simulink model "leg"  (R2024a)
settings: Solver=ode15s  StartTime=0.0  StopTime=11  FixedStep=0.1  RelTol=1e-3
values from neighbouring files (symbols this model uses):
  m = RIGHT_LEG(joint_name).m    [test_dynamics.m]
  motion_time_constant = 1e-3    (= 0.001)    [Initialization.m]
undefined symbols (not defined in the file or in its folder): LEFT_LEG_FEEDBACK_GAIN, RIGHT_LEG_FEEDBACK_GAIN, X, Y, Z
libraries: sm_lib x104, nesl_utility x35, slpidlib x20
(part 1 of 5)
settings Model: Creator=daniel  LastModifiedBy=daniel

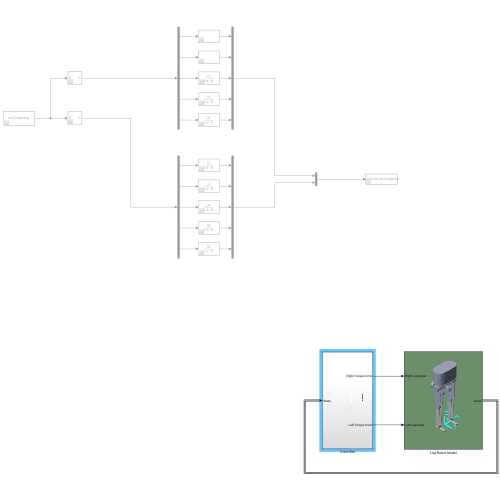
[thumbnail: Simulink's stored preview of the top-level diagram]
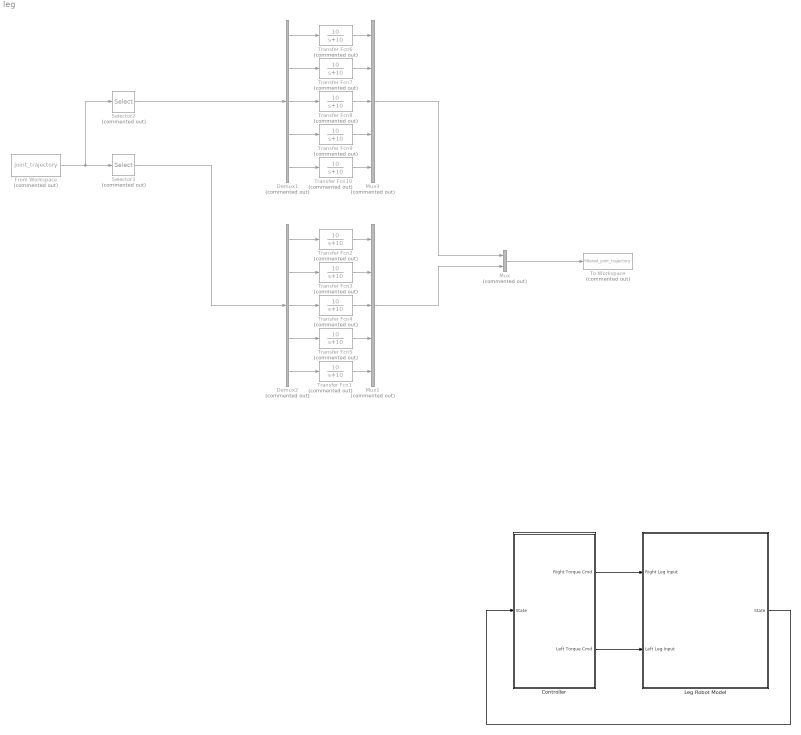
== system leg ==
  Controller : Subsystem
  Demux1 : Demux  Commented=on  Outputs=5
  Demux2 : Demux  Commented=on  Outputs=5
  From Workspace : FromWorkspace  Commented=on  VariableName=joint_trajectory
  Leg Robot Model : Subsystem
      mask Display: image('leg_robot.png');
  Mux : Mux  Commented=on  Inputs=2
  Mux1 : Mux  Commented=on  Inputs=5
  Mux3 : Mux  Commented=on  Inputs=5
  Selector2 : Selector  Commented=on  InputPortWidth=10  IndexOptions=Index vector (dialog)  Indices=[1:5]  OutputSizes=1
  Selector3 : Selector  Commented=on  InputPortWidth=10  IndexOptions=Index vector (dialog)  Indices=[6:10]  OutputSizes=1
  To Workspace : ToWorkspace  Commented=on  VariableName=filtered_joint_trajectory  SaveFormat=Structure With Time  SampleTime=-1
  Transfer Fcn{1..10} (10 alike) : TransferFcn  Commented=on  Numerator=[10]  Denominator=[1 10]
  wires:
  Controller/1(Right Torque Cmd) -> Leg Robot Model/1(Right Leg Input)
  Controller/2(Left Torque Cmd) -> Leg Robot Model/2(Left Leg Input)
  Leg Robot Model/1(State) -> Controller/1(State)
  Transfer Fcn10/1 -> Mux3/5
  Demux1/5 -> Transfer Fcn10/1
  Demux1/3 -> Transfer Fcn8/1
  Transfer Fcn6/1 -> Mux3/1
  Demux1/4 -> Transfer Fcn9/1
  Transfer Fcn8/1 -> Mux3/3
  Transfer Fcn7/1 -> Mux3/2
  Transfer Fcn9/1 -> Mux3/4
  Demux1/1 -> Transfer Fcn6/1
  Demux1/2 -> Transfer Fcn7/1
  From Workspace/1 -> Selector2/1, Selector3/1
  Selector2/1 -> Demux1/1
  Selector3/1 -> Demux2/1
  Transfer Fcn4/1 -> Mux1/3
  Transfer Fcn2/1 -> Mux1/1
  Demux2/5 -> Transfer Fcn1/1
  Transfer Fcn3/1 -> Mux1/2
  Demux2/2 -> Transfer Fcn3/1
  Mux1/1 -> Mux/2
  Demux2/4 -> Transfer Fcn5/1
  Transfer Fcn5/1 -> Mux1/4
  Demux2/1 -> Transfer Fcn2/1
  Demux2/3 -> Transfer Fcn4/1
  Transfer Fcn1/1 -> Mux1/5
  Mux/1 -> To Workspace/1
  Mux3/1 -> Mux/1

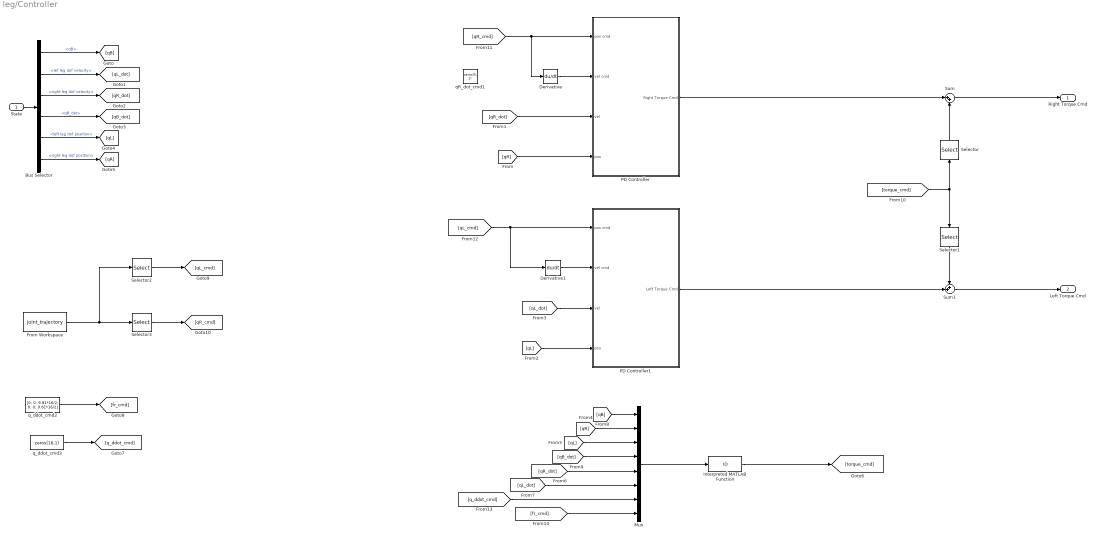
== system leg/Controller ==
  State : Inport
  Bus Selector : BusSelector  OutputSignals=qB,lef leg dof velocity,right leg dof velocity,qB_dot,left leg dof position,right leg dof position
  Derivative : Derivative  CoefficientInTFapproximation=0
  Derivative1 : Derivative  CoefficientInTFapproximation=0
  From Workspace : FromWorkspace  VariableName=joint_trajectory
  Interpreted MATLAB Function : MATLABFcn  MATLABFcn=ID
  Mux : Mux  Inputs=8
  PD Controller : Subsystem
  PD Controller1 : Subsystem
  Selector : Selector  InputPortWidth=10  IndexOptions=Index vector (dialog)  Indices=[1:5]  OutputSizes=1
  Selector1 : Selector  InputPortWidth=10  IndexOptions=Index vector (dialog)  Indices=[6:10]  OutputSizes=1
  Selector2 : Selector  InputPortWidth=10  IndexOptions=Index vector (dialog)  Indices=[1:5]  OutputSizes=1
  Selector3 : Selector  InputPortWidth=10  IndexOptions=Index vector (dialog)  Indices=[6:10]  OutputSizes=1
  Sum : Sum  Inputs=|++
  Sum1 : Sum  Inputs=++|
  qR_dot_cmd1 : Constant  Value=zeros(5, 1)
  q_ddot_cmd2 : Constant  Value=[0; 0; 9.81*16/2; 0; 0; 9.81*16/2]
  q_ddot_cmd3 : Constant  Value=zeros(16,1)
  Right Torque Cmd : Outport
  Left Torque Cmd : Outport  Port=2
  wires:
  State/1 -> Bus Selector/1
  Bus Selector/1 -> [qB]  "<qB>"
  Bus Selector/2 -> [qL_dot]  "<lef leg dof velocity>"
  Bus Selector/3 -> [qR_dot]  "<right leg dof velocity>"
  Bus Selector/4 -> [qB_dot]  "<qB_dot>"
  Bus Selector/5 -> [qL]  "<left leg dof position>"
  Bus Selector/6 -> [qR]  "<right leg dof position>"
  [qR] -> PD Controller/4(pos)
  [qR_dot] -> PD Controller/3("vel ")
  [qL] -> PD Controller1/4(pos)
  [qL_dot] -> PD Controller1/3("vel ")
  PD Controller/1(Right Torque Cmd) -> Sum/1
  Sum/1 -> Right Torque Cmd/1
  Sum1/1 -> Left Torque Cmd/1
  PD Controller1/1(Left Torque Cmd) -> Sum1/2
  Selector/1 -> Sum/2
  Selector1/1 -> Sum1/1
  [q_ddot_cmd] -> Mux/7
  [qL] -> Mux/3
  [qR] -> Mux/2
  [qL_dot] -> Mux/6
  [qR_dot] -> Mux/5
  [qB] -> Mux/1
  [qB_dot] -> Mux/4
  [fr_cmd] -> Mux/8
  [torque_cmd] -> Selector1/1, Selector/1
  Mux/1 -> Interpreted MATLAB Function/1
  From Workspace/1 -> Selector3/1, Selector2/1
  Selector2/1 -> [qL_cmd]
  Selector3/1 -> [qR_cmd]
  q_ddot_cmd2/1 -> [fr_cmd]
  q_ddot_cmd3/1 -> [q_ddot_cmd]
  Derivative/1 -> PD Controller/2(vel cmd)
  Derivative1/1 -> PD Controller1/2(vel cmd)
  Interpreted MATLAB Function/1 -> [torque_cmd]
  [qL_cmd] -> Derivative1/1, PD Controller1/1(pos cmd)
  [qR_cmd] -> Derivative/1, PD Controller/1(pos cmd)

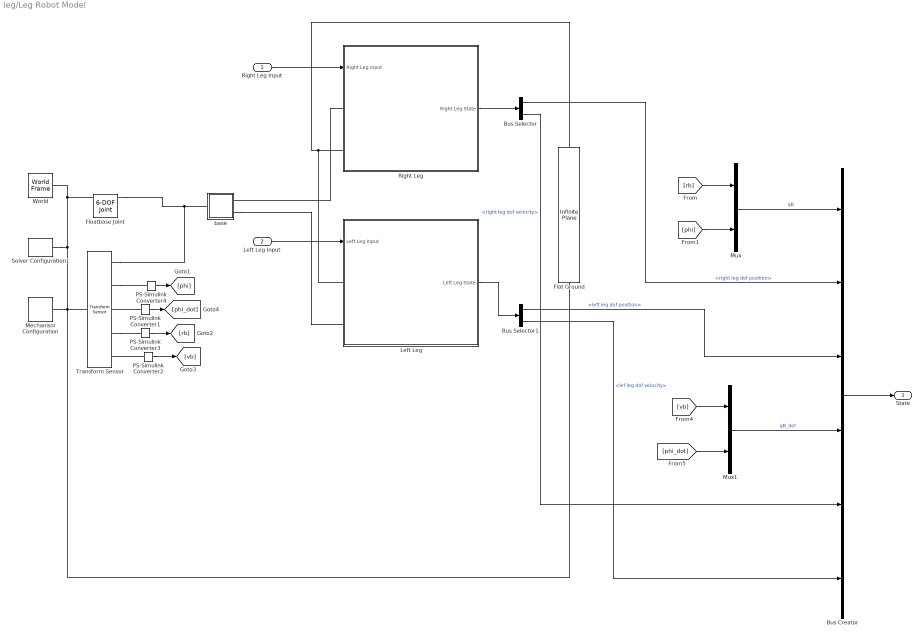
== system leg/Leg Robot Model ==
  Right Leg Input : Inport
  Left Leg Input : Inport  Port=2
  Bus Creator : BusCreator  Inputs=6
  Bus Selector : BusSelector  OutputSignals=right leg dof position,right leg dof velocity
  Bus Selector1 : BusSelector  OutputSignals=left leg dof position,lef leg dof velocity
  Flat Ground : sm_lib/Curves and Surfaces/Infinite Plane  GraphicType=Rectangle  GraphicPlaneWidth=5  GraphicPlaneWidthUnits=m  GraphicPlaneHeight=5  GraphicPlaneHeightUnits=m  GraphicVisPropType=SimpleVisualProperties  GraphicDiffuseColor=[0.07451 0.6235 1]  GraphicOpacity=0.75  GraphicSpecularColor=[0.5 0.5 0.5 1.0]  GraphicAmbientColor=[0.15 0.15 0.15 1.0]  GraphicEmissiveColor=[0.0 0.0 0.0 1.0]  GraphicShininess=75
  Floatbase Joint : sm_lib/Joints/6-DOF Joint  JointMode=Normal  CompositeWrenchDir=FollowerOnBase  CompositeWrenchFrame=BaseFrame  SenseConstraintForce=off  SenseConstraintTorque=off  SenseTotalForce=off  SenseTotalTorque=off  PxPositionTargetSpecify=on  PxPositionTargetPriority=High  PxPositionTargetValue=0  PxPositionTargetValueUnits=m  PxVelocityTargetSpecify=on  PxVelocityTargetPriority=High  PxVelocityTargetValue=0  PxVelocityTargetValueUnits=m/s  PxEquilibriumPosition=0  PxEquilibriumPositionUnits=m  PxSpringStiffness=0  PxSpringStiffnessUnits=N/m  PxDampingCoefficient=0.001  PxDampingCoefficientUnits=N/(m/s)  PxLowerLimitSpecify=off  PxLowerLimitBound=-1  PxLowerLimitBoundUnits=m  PxLowerLimitStiffness=1e6  PxLowerLimitStiffnessUnits=N/m  PxLowerLimitDamping=1e3  PxLowerLimitDampingUnits=N/(m/s)  PxLowerLimitTransitionRegionWidth=1e-4  PxLowerLimitTransitionRegionWidthUnits=m  PxUpperLimitSpecify=off  PxUpperLimitBound=1  PxUpperLimitBoundUnits=m  PxUpperLimitStiffness=1e6  PxUpperLimitStiffnessUnits=N/m  PxUpperLimitDamping=1e3  PxUpperLimitDampingUnits=N/(m/s)  PxUpperLimitTransitionRegionWidth=1e-4  PxUpperLimitTransitionRegionWidthUnits=m  PxTorqueActuationMode=InputTorque  PxMotionActuationMode=ComputedMotion  PxSensePosition=off  PxSenseVelocity=off  PxSenseAcceleration=off  PxSenseTorqueForce=off  PxSenseLowerLimitTorqueForce=off  PxSenseUpperLimitTorqueForce=off  PyPositionTargetSpecify=on  PyPositionTargetPriority=High  PyPositionTargetValue=0  PyPositionTargetValueUnits=m  PyVelocityTargetSpecify=on  PyVelocityTargetPriority=High  PyVelocityTargetValue=0  PyVelocityTargetValueUnits=m/s  PyEquilibriumPosition=0  PyEquilibriumPositionUnits=m  PySpringStiffness=0  PySpringStiffnessUnits=N/m  PyDampingCoefficient=0.001  PyDampingCoefficientUnits=N/(m/s)  PyLowerLimitSpecify=off  PyLowerLimitBound=-1  PyLowerLimitBoundUnits=m  PyLowerLimitStiffness=1e6  PyLowerLimitStiffnessUnits=N/m  PyLowerLimitDamping=1e3  PyLowerLimitDampingUnits=N/(m/s)  PyLowerLimitTransitionRegionWidth=1e-4  PyLowerLimitTransitionRegionWidthUnits=m  PyUpperLimitSpecify=off  PyUpperLimitBound=1  PyUpperLimitBoundUnits=m  PyUpperLimitStiffness=1e6  PyUpperLimitStiffnessUnits=N/m  PyUpperLimitDamping=1e3  PyUpperLimitDampingUnits=N/(m/s)  PyUpperLimitTransitionRegionWidth=1e-4  PyUpperLimitTransitionRegionWidthUnits=m  PyTorqueActuationMode=InputTorque  PyMotionActuationMode=ComputedMotion  PySensePosition=off  PySenseVelocity=off  PySenseAcceleration=off  PySenseTorqueForce=off  PySenseLowerLimitTorqueForce=off  PySenseUpperLimitTorqueForce=off  PzPositionTargetSpecify=on  PzPositionTargetPriority=High  PzPositionTargetValue=0.862  PzPositionTargetValueUnits=m  PzVelocityTargetSpecify=off  PzVelocityTargetPriority=High  PzVelocityTargetValue=0  PzVelocityTargetValueUnits=m/s  PzEquilibriumPosition=0  PzEquilibriumPositionUnits=m  PzSpringStiffness=0  PzSpringStiffnessUnits=N/m  PzDampingCoefficient=0.001  PzDampingCoefficientUnits=N/(m/s)  PzLowerLimitSpecify=off  PzLowerLimitBound=-1  PzLowerLimitBoundUnits=m  PzLowerLimitStiffness=1e6  PzLowerLimitStiffnessUnits=N/m  PzLowerLimitDamping=1e3  PzLowerLimitDampingUnits=N/(m/s)  PzLowerLimitTransitionRegionWidth=1e-4  PzLowerLimitTransitionRegionWidthUnits=m  PzUpperLimitSpecify=off  PzUpperLimitBound=1  PzUpperLimitBoundUnits=m  PzUpperLimitStiffness=1e6  PzUpperLimitStiffnessUnits=N/m  PzUpperLimitDamping=1e3  PzUpperLimitDampingUnits=N/(m/s)  PzUpperLimitTransitionRegionWidth=1e-4  PzUpperLimitTransitionRegionWidthUnits=m  PzTorqueActuationMode=NoTorque  PzMotionActuationMode=ComputedMotion  PzSensePosition=off  PzSenseVelocity=off  PzSenseAcceleration=off  PzSenseTorqueForce=off  PzSenseLowerLimitTorqueForce=off  PzSenseUpperLimitTorqueForce=off  SphPositionTargetSpecify=on  SphPositionTargetPriority=High  SphPositionTargetRotationMethod=RotationSequence  SphPositionTargetFollAlignAxisA=+X  SphPositionTargetBaseAlignAxisA=+Y  SphPositionTargetFollAlignAxisB=+Y  SphPositionTargetBaseAlignAxisB=+Z  SphPositionTargetRotationStandardAxis=+Y  SphPositionTargetRotationAngle=10  SphPositionTargetRotationAngleUnits=deg  SphPositionTargetRotationArbitraryAxis=[0 0 1]  SphPositionTargetRotationSequenceAxes=BaseAxes  SphPositionTargetRotationSequence=XYZ  SphPositionTargetRotationSequenceAngles=[0 0 0]  SphPositionTargetRotationSequenceAnglesUnits=deg  SphPositionTargetRotationMatrix=[1 0 0; 0 1 0; 0 0 1]  SphPositionTargetQuaternion=[1 0 0 0]  SphVelocityTargetSpecify=off  SphVelocityTargetPriority=High  SphVelocityTargetValue=[0 0 0]  SphVelocityTargetValueUnits=deg/s  SphVelocityTargetInFollowerFrame=on  SphEqPosRotationMethod=None  SphEqPosFollAlignAxisA=+X  SphEqPosBaseAlignAxisA=+Y  SphEqPosFollAlignAxisB=+Y  SphEqPosBaseAlignAxisB=+Z  SphEqPosRotationStandardAxis=+Z  SphEqPosRotationAngle=0.0  SphEqPosRotationAngleUnits=deg  SphEqPosRotationArbitraryAxis=[0 0 1]  SphEqPosRotationSequenceAxes=FollowerAxes  SphEqPosRotationSequence=XYX  SphEqPosRotationSequenceAngles=[0 0 0]  SphEqPosRotationSequenceAnglesUnits=deg  SphEqPosRotationMatrix=[1 0 0; 0 1 0; 0 0 1]  SphEqPosQuaternion=[1 0 0 0]  SphSpringStiffness=0  SphSpringStiffnessUnits=N*m/deg  SphDampingCoefficient=1e-3  SphDampingCoefficientUnits=N*m/(rad/s)  SphLowerLimitSpecify=off  SphLowerLimitBound=15  SphLowerLimitBoundUnits=deg  SphLowerLimitStiffness=1e4  SphLowerLimitStiffnessUnits=N*m/deg  SphLowerLimitDamping=10  SphLowerLimitDampingUnits=N*m/(deg/s)  SphLowerLimitTransitionRegionWidth=0.1  SphLowerLimitTransitionRegionWidthUnits=deg  SphUpperLimitSpecify=off  SphUpperLimitBound=45  SphUpperLimitBoundUnits=deg  SphUpperLimitStiffness=1e4  SphUpperLimitStiffnessUnits=N*m/deg  SphUpperLimitDamping=10  SphUpperLimitDampingUnits=N*m/(deg/s)  SphUpperLimitTransitionRegionWidth=0.1  SphUpperLimitTransitionRegionWidthUnits=deg  SphTorqueActuationMode=NoTorque  SphActuateTorqueX=off  SphActuateTorqueY=off  SphActuateTorqueZ=off  SphActuateTorque=off  SphActuationFrame=BaseFrame  SphSensePosition=on  SphSenseVelocityX=off  SphSenseVelocityY=off  SphSenseVelocityZ=off  SphSenseVelocity=on  SphSenseAccelerationX=off  SphSenseAccelerationY=off  SphSenseAccelerationZ=off  SphSenseAcceleration=off  SphSenseLowerLimitTorqueMag=off  SphSenseUpperLimitTorqueMag=off  SphSensingFrame=BaseFrame
  Left Leg : Subsystem
  Mechanism Configuration : sm_lib/Utilities/Mechanism Configuration  UniformGravity=Constant  GravityVector=[0 0 -9.80665]  GravityVectorUnits=m/s^2  LinearizationDelta=0.001  JointModeTransitionNonlinearIterations=2
  Mux : Mux  Inputs=2
  Mux1 : Mux  Inputs=2
  PS-Simulink Converter{1..4} (4 alike) : nesl_utility/PS-Simulink Converter  PhysicalDomain=network_engine_domain  SubClassName=ps_output  LeftPortType=input  RightPortType=output  PseudoPeriodic=off  Frequencies=[]  VectorFormat=inherit  Unit=inherit  AffineConversion=off
  Right Leg : Subsystem
  Solver Configuration1 : nesl_utility/Solver Configuration  PhysicalDomain=network_engine_domain  SubClassName=solver  LeftPortType=input  RightPortType=generic  Tones=[]  Harmonics=[]  SimulateNoise=off  Profile=off  UseLocalSampling=off  EnableSwitchedLinearOptims=on  FrequencyDomain=off  UseCCode=off  RelTol=0.001  AbsTol=1e-06  MinStep=1e-09  ToWorkspace=off  RevertToSquareIcSolve=off  NumHomotopyIterations=100  PhasorMode=off  PhasorModeNumHarmonics=1  ConsistencySolver=NEWTON_FTOL  IndexReductionMethod=DerivativeReplacement  DoDC=off  ResidualTolerance=1e-09  ConsistencyTolSource=GLOBAL  ConsistencyAbsTol=0.001  ConsistencyRelTol=0.001  ConsistencyTolFactor=0.001  UseLocalSolver=off  LocalSolverChoice=NE_BACKWARD_EULER_ADVANCER  ResolveIndetEquations=on  FunctionEvalNumThread=1  LocalSolverSampleTime=0.001  DoFixedCost=off  MaxNonlinIter=3  MaxModeIter=2  ComputeImpulses=off  ImpulseIterations=2  LinearAlgebra=Sparse  LinearAlgebraNumThread=0  EquationFormulation=NE_TIME_EF  DelaysMemoryBudget=1024  AutomaticFiltering=on  FilteringTimeConstant=0.001  PartitionStorageMethod=AS_NEEDED  PartitionMemoryBudget=1024  PartitionMethod=FAST  MultibodyUseLocalSolver=off  MultibodyLocalSolverChoice=ODE1  MultibodyLocalSolverSampleTime=0.001
  Transform Sensor : sm_lib/Frames and Transforms/Transform Sensor  MeasurementFrame=World  RotationSequence=XYZ  SenseAngle=off  SenseAxis=off  SenseQ=off  SenseR=off  SenseRotationSequence=on  SenseOmegaX=off  SenseOmegaY=off  SenseOmegaZ=off  SenseOmega=off  SenseQDot=off  SenseRDot=off  SenseRotationSequenceDot=on  SenseAlphaX=off  SenseAlphaY=off  SenseAlphaZ=off  SenseAlpha=off  SenseQDDot=off  SenseRDDot=off  SenseX=off  SenseY=off  SenseZ=off  SenseXYZ=on  SenseRad=off  SenseAzim=off  SenseDist=off  SenseInc=off  SenseXDot=off  SenseYDot=off  SenseZDot=off  SenseXYZDot=on  SenseRadDot=off  SenseAzimDot=off  SenseDistDot=off  SenseIncDot=off  SenseXDDot=off  SenseYDDot=off  SenseZDDot=off  SenseXYZDDot=off  SenseRadDDot=off  SenseAzimDDot=off  SenseDistDDot=off  SenseIncDDot=off
  World : sm_lib/Frames and Transforms/World Frame
  base : Subsystem
  State : Outport
  wires:
  PS-Simulink Converter3/1 -> [rb]
  PS-Simulink Converter2/1 -> [vb]
  PS-Simulink Converter1/1 -> [phi_dot]
  PS-Simulink Converter4/1 -> [phi]
  Right Leg Input/1 -> Right Leg/1(Right Leg Input)
  Left Leg Input/1 -> Left Leg/1(Left Leg Input)
  [rb] -> Mux/1
  [phi] -> Mux/2
  Mux/1 -> Bus Creator/1  "qB"
  Bus Selector/1 -> Bus Creator/2  "<right leg dof position>"
  Mux1/1 -> Bus Creator/4  "qB_dot"
  [phi_dot] -> Mux1/2
  [vb] -> Mux1/1
  Right Leg/1(Right Leg State) -> Bus Selector/1
  Left Leg/1(Left Leg State) -> Bus Selector1/1
  Bus Selector1/1 -> Bus Creator/3  "<left leg dof position>"
  Bus Selector/2 -> Bus Creator/5  "<right leg dof velocity>"
  Bus Selector1/2 -> Bus Creator/6  "<lef leg dof velocity>"
  Bus Creator/1 -> State/1
  connections:
  Mechanism Configuration/RConn1 -- Flat Ground/LConn1 -- Transform Sensor/LConn1 -- Solver Configuration1/RConn1 -- Floatbase Joint/LConn1 -- World/RConn1
  Right Leg/LConn1 -- base/RConn1
  Right Leg/LConn2 -- Left Leg/LConn1 -- Flat Ground/RConn1
  PS-Simulink Converter2/LConn1 -- Transform Sensor/RConn5
  Transform Sensor/RConn4 -- PS-Simulink Converter3/LConn1
  Transform Sensor/RConn2 -- PS-Simulink Converter4/LConn1
  PS-Simulink Converter1/LConn1 -- Transform Sensor/RConn3
  base/RConn2 -- Left Leg/LConn2
  Floatbase Joint/RConn1 -- Transform Sensor/RConn1 -- base/LConn1
